simulink model "ConvertPIDTodDec"  (R2021b)
settings: Solver=FixedStepAuto  StartTime=0.0  StopTime=10.0  FixedStep=0.2  RelTol=1e-3
libraries: simulink x1
settings Model: Creator=ajfem  LastModifiedBy=ajfem

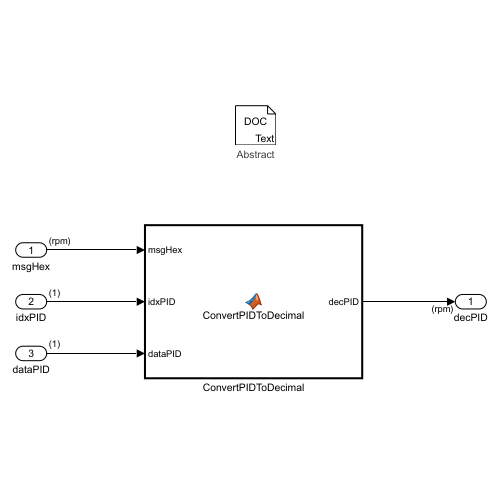
[thumbnail: Simulink's stored preview of the top-level diagram]
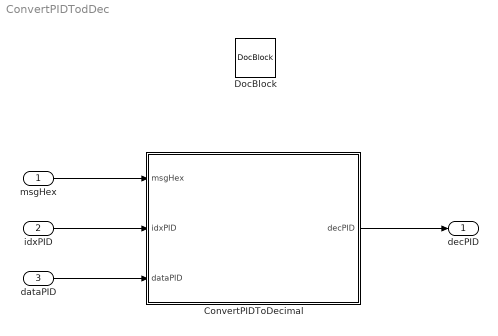
== system ConvertPIDTodDec ==
  msgHex : Inport  OutDataTypeStr=double  Unit=rpm  PortDimensions=1
  idxPID : Inport  Port=2  OutDataTypeStr=uint8  Unit=1  PortDimensions=1
  dataPID : Inport  Port=3  OutDataTypeStr=uint8  Unit=1  PortDimensions=1
  ConvertPIDToDecimal : MATLAB Function  TreatAsAtomicUnit=on
  DocBlock : simulink/Model-Wide Utilities/DocBlock  ECoderFlag=Abstract  DocumentType=Text
      content=|
      | This model converts rpm hex values to rpm decimal values.
      settings: AttributesFormatString=%<ECoderFlag>
  decPID : Outport  OutDataTypeStr=double  Unit=rpm  PortDimensions=1
  wires:
  msgHex/1 -> ConvertPIDToDecimal/1(msgHex)
  idxPID/1 -> ConvertPIDToDecimal/2(idxPID)
  ConvertPIDToDecimal/1(decPID) -> decPID/1
  dataPID/1 -> ConvertPIDToDecimal/3(dataPID)

== matlab function ConvertPIDTodDec/ConvertPIDToDecimal ==
  data: msgHex input; decPID output double size=1; idxPID input uint8 size=1; dataPID input uint8 size=1
function decPID = ConvertPIDToDecimal(msgHex, idxPID, dataPID)
%#codegen

decPID = msgHex;
